simulink model "PalmSatKalman"  (R2017b)
settings: Solver=VariableStepAuto  StartTime=0.0  StopTime=10.0  RelTol=1e-3
values from neighbouring files (symbols this model uses):
  A = ModeloSatelite.A    [PalmSatModelScript.m]
  B = ModeloSatelite.B    [PalmSatModelScript.m]
  C = ModeloSatelite.C    [PalmSatModelScript.m]
  cimotor_11 = 0    [PalmSatModelScript.m]
  cimotor_12 = 0    [PalmSatModelScript.m]
  cimotor_13 = 0    [PalmSatModelScript.m]
  cimotor_14 = 0    [PalmSatModelScript.m]
  ciobserv_11 = 0    [PalmSatModelScript.m]
  ciobserv_12 = 0    [PalmSatModelScript.m]
  ciobserv_13 = 0    [PalmSatModelScript.m]
  ciobserv_14 = 0    [PalmSatModelScript.m]
  D = ModeloSatelite.D    [PalmSatModelScript.m]
  F = inv(G)    [PalmSatModelScript.m]
  L = S*C'*inv(rv)    [PalmSatModelScript.m]
undefined symbols (not defined in the file or in its folder): kc
settings Model: Creator=Gpiaia  LastModifiedBy=Gpiaia

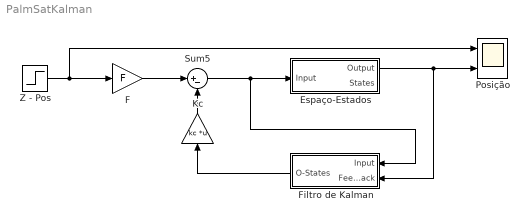
== system PalmSatKalman ==
  Espaço-Estados : Subsystem
  F : Gain  Gain=F
  Filtro de Kalman : Subsystem
  Kc : Gain  Gain=kc  Multiplication=Matrix(K*u)
  Posição : Scope  NumInputPorts=2
  Sum5 : Sum  Inputs=|+-
  Z - Pos : Step  Time=0.5  After=45  SampleTime=0  VectorParams1D=off
  wires:
  Z - Pos/1 -> F/1, Posição/1
  Filtro de Kalman/1(O-States) -> Kc/1
  F/1 -> Sum5/1
  Kc/1 -> Sum5/2
  Espaço-Estados/1(Output) -> Posição/2, Filtro de Kalman/2(Feedback)
  Sum5/1 -> Filtro de Kalman/1(Input), Espaço-Estados/1(Input)

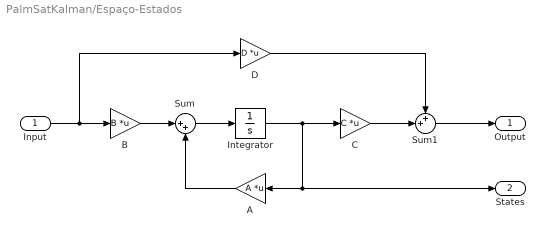
== system PalmSatKalman/Espaço-Estados ==
  Input : Inport
  A : Gain  Gain=A  Multiplication=Matrix(K*u)
  B : Gain  Gain=B  Multiplication=Matrix(K*u)
  C : Gain  Gain=C  Multiplication=Matrix(K*u)
  D : Gain  Gain=D  Multiplication=Matrix(K*u)
  Integrator : Integrator  InitialCondition=[cimotor_11; cimotor_12; cimotor_13; cimotor_14]
  Sum : Sum  Inputs=|++
  Sum1 : Sum  Inputs=++|
  Output : Outport
  States : Outport  Port=2
  wires:
  Sum1/1 -> Output/1
  Integrator/1 -> A/1, States/1, C/1
  A/1 -> Sum/2
  D/1 -> Sum1/1
  B/1 -> Sum/1
  Sum/1 -> Integrator/1
  C/1 -> Sum1/2
  Input/1 -> D/1, B/1

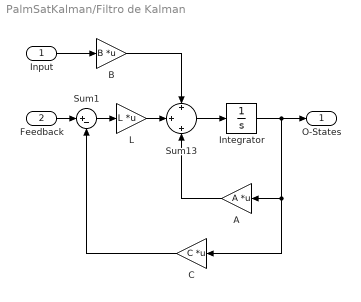
== system PalmSatKalman/Filtro de Kalman ==
  Input : Inport
  Feedback : Inport  Port=2
  A : Gain  Gain=A  Multiplication=Matrix(K*u)  SaturateOnIntegerOverflow=on  OutDataTypeStr=Inherit: Same as input  ParamDataTypeStr=Inherit: Same as input
  B : Gain  Gain=B  Multiplication=Matrix(K*u)  SaturateOnIntegerOverflow=on  OutDataTypeStr=Inherit: Same as input  ParamDataTypeStr=Inherit: Same as input
  C : Gain  Gain=C  Multiplication=Matrix(K*u)  SaturateOnIntegerOverflow=on  OutDataTypeStr=Inherit: Same as input  ParamDataTypeStr=Inherit: Same as input
  Integrator : Integrator  InitialCondition=[ciobserv_11; ciobserv_12; ciobserv_13; ciobserv_14]
  L : Gain  Gain=L  Multiplication=Matrix(K*u)  SaturateOnIntegerOverflow=on  OutDataTypeStr=Inherit: Same as input  ParamDataTypeStr=Inherit: Same as input
  Sum1 : Sum  Inputs=|+-  SaturateOnIntegerOverflow=on  InputSameDT=on  OutDataTypeStr=Inherit: Same as first input
  Sum13 : Sum  Inputs=+|+|+  SaturateOnIntegerOverflow=on  InputSameDT=on  OutDataTypeStr=Inherit: Same as first input
  O-States : Outport
  wires:
  Input/1 -> B/1
  Integrator/1 -> O-States/1, A/1, C/1
  Sum13/1 -> Integrator/1
  A/1 -> Sum13/3
  B/1 -> Sum13/1
  L/1 -> Sum13/2
  Sum1/1 -> L/1
  Feedback/1 -> Sum1/1
  C/1 -> Sum1/2
